simulink model "Factorial"  (R2021a)
settings: Solver=VariableStepAuto  StartTime=0.0  StopTime=10.0  RelTol=1e-3
settings Model: Creator=Moamen_Hamed  LastModifiedBy=Moamen_Hamed

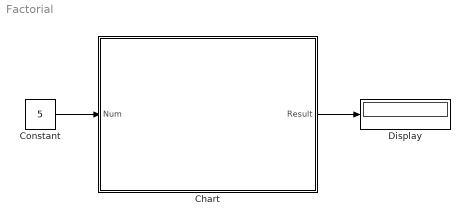
== system Factorial ==
  Chart : Stateflow chart  TreatAsAtomicUnit=on
  Constant : Constant  Value=5
  Display : Display
  wires:
  Constant/1 -> Chart/1(Num)
  Chart/1(Result) -> Display/1

== stateflow chart Factorial/Chart ==
  (default) -> (junction 13)
  (junction 13) -> (junction 15) : {Result = 1;Temp = Num;}
  (junction 15) -> (junction 14) [order 1] : [Temp > 1]
  (junction 16) -> (junction 15)
  (junction 14) -> (junction 16) : { Result = Result * Temp;Temp = Temp - 1;}
  (junction 15) -> (junction 17) [order 2]
  data: Num input; Result output; Temp local
